simulink library "dspmathops"  (Simulink 8.0)
settings: Solver=ode45  SolverMode=SingleTasking  StartTime=0.0  StopTime=10.0  RelTol=1e-3
values from neighbouring files (symbols this model uses):
  D = D + B    [rebuffer_delay.m]
undefined symbols (not defined in the file or in its folder): dBval, Floor, fuzz_val, jsin, magnitude
libraries: dspsigattribs x2
settings Model: RequirementInfo=9  Creator=don  LastModifiedBy=lij  CovMetricSettings=d  ExtModeAutoUpdateStatusClock=off

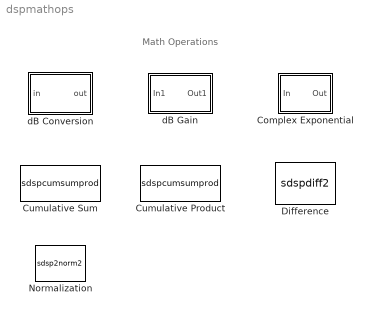
== system dspmathops ==
  note: Math Operations
  Complex Exponential : Subsystem
      mask Type: Complex Exponential
      mask Description:
      | Compute the complex exponential function of real inputs via
      | Euler's formula, y = cos(x)+jsin(x).
      mask Help: eval('blocksethelp');
      mask Display: text(0.2, 0.55,'exp(jx)');
  Cumulative Product : S-Function  DialogController=dspDDGCreate  DialogControllerArgs=DataTag1  FunctionName=sdspcumsumprod  Parameters=dim,InputProcessing,reset,fcn,outputMin,outputMax,dtInfo.interProdMode,dtInfo.interProdWordLength,dtInfo.interProdFracLength,dtInfo.prodOutputMode,dtInfo.prodOutputWordLength,dtInfo.prodOutputFracLength,dtInfo.accumMode,dtInfo.accumWordLength,dtInfo.accumFracLength,dtInfo.outputMode,dtInfo.outputWordLength,dtInfo.outputFracLength,dtInfo.roundingMode,dtInfo.overflowMode  EnableBusSupport=off  mask(Cumulative Product){dim=Channels (running product), InputProcessing=Columns as channels (frame based), reset_popup=None, interProdMode=Same as input, interProdWordLength=16, interProdFracLength=15, interProdDataTypeStr=Inherit: Same as input, interProdLastDataTypeStr=Inherit: Same as input, prodOutputMode=Same as input, prodOutputWordLength=32, prodOutputFracLength=30, prodOutputDataTypeStr=Inherit: Same as input, prodOutputLastDataTypeStr=Inherit: Same as input, accumMode=Same as input, accumWordLength=32, accumFracLength=30, accumDataTypeStr=Inherit: Same as input, accumLastDataTypeStr=Inherit: Same as input, outputMode=Same as input, outputWordLength=16, outputFracLength=15, outputDataTypeStr=Inherit: Same as input, outputLastDataTypeStr=Inherit: Same as input, outputMin=[], outputMax=[], roundingMode=Floor, overflowMode=off, LockScale=off}
      mask prompts: dim "Multiply input along:"; InputProcessing "Input processing:"; reset_popup "Reset port:"; interProdMode "inter prod mode"; interProdWordLength "inter prod wl"; interProdFracLength "inter prod fl"; interProdDataTypeStr "Intermediate product data type string:"; interProdLastDataTypeStr "Last intermediate product data type string:"; prodOutputMode "prod output mode"; prodOutputWordLength "prod output wl"; prodOutputFracLength "prod output fl"; prodOutputDataTypeStr "ProdOutput data type string:"; prodOutputLastDataTypeStr "Last prodOutput data type string:"; accumMode "accum mode"; accumWordLength "accum wl"; accumFracLength "accum fl"; accumDataTypeStr "Accum data type string:"; accumLastDataTypeStr "Last accum data type string:"; outputMode "output mode"; outputWordLength "output wl"; outputFracLength "output fl"; outputDataTypeStr "Output data type string:"; outputLastDataTypeStr "Last output data type string:"; outputMin "Output minimum:"; outputMax "Output maximum:"; roundingMode "rm"; overflowMode "om"; LockScale "Lock scaling"
      mask help: Cumulative product of input matrix or input vector elements along the specified dimension: rows, columns, or channels.
      mask init:
      | blkh   = gcbh;
      | reset  = reset_popup-1;
      | fcn    = 1;
      | dspSetFrameUpgradeParameter(blkh, 'InputProcessing', 'Inherited (this choice will be removed - see release notes)');
      | dtRows = dspblkGetCumProdDTRowInfo();
      | dtInfo = dspGetUDTFixptDataTypeInfo(blkh, dtRows, true);
      mask Help: eval('blocksethelp');
      mask StyleString: popup(Columns|Rows|Channels (running product)),popup(Columns as channels (frame based)|Elements as channels (sample based)|Inherited (this choice will be removed - see release notes)),popup(None|Rising edge|Falling edge|Either edge|Non-zero sample),popup(Same as input|Binary point scaling|Slope and bias scaling),edit,edit,unidt({a=7|||}{i=Inherit: Same as input}{s=UDTBinaryPointMode}{g=UDTInheritSign}),edit,popup(Same as input|Binary point scaling|Slope and bias scaling),edit,edit,unidt({a=12|||}{i=Inherit: Same as input}{s=UDTBinaryPointMode}{g=UDTInheritSign}),edit,popup(Same as product output|Same as input|Binary point scaling|Slope and bias scaling),edit,edit,unidt({a=17|||}{i=Inherit: Same as input|Inherit: Same as product output}{s=UDTBinaryPointMode}{g=UDTInheritSign}),edit,popup(Same as product output|Same as input|Binary point scaling|Slope and bias scaling),edit,edit,unidt({a=22|24|25|}{i=Inherit: Same as input|Inherit: Same as product output}{s=UDTBinaryPointMode}{g=UDTInheritSign}),edit,min,max,popup(Ceiling|Convergent|Floor|Nearest|Round|Simplest|Zero),checkbox,checkbox
      mask Display:
      | s = dspblkcumsumprod();
      | disp([s.str '\nProduct'])
      | port_label('input',s.i1,s.i1s);
      | port_label('input',s.i2,s.i2s);
  Cumulative Sum : S-Function  DialogController=dspDDGCreate  DialogControllerArgs=DataTag3  FunctionName=sdspcumsumprod  Parameters=dim,InputProcessing,reset,fcn,outputMin,outputMax,-1,0,0,-1,0,0,dtInfo.accumMode,dtInfo.accumWordLength,dtInfo.accumFracLength,dtInfo.outputMode,dtInfo.outputWordLength,dtInfo.outputFracLength,dtInfo.roundingMode,dtInfo.overflowMode  EnableBusSupport=off  mask(Cumulative Sum){dim=Channels (running sum), InputProcessing=Columns as channels (frame based), reset_popup=None, accumMode=Same as input, accumWordLength=32, accumFracLength=30, accumDataTypeStr=Inherit: Same as input, accumLastDataTypeStr=Inherit: Same as input, outputMode=Same as accumulator, outputWordLength=16, outputFracLength=15, outputDataTypeStr=Inherit: Same as accumulator, outputLastDataTypeStr=Inherit: Same as accumulator, outputMin=[], outputMax=[], roundingMode=Floor, overflowMode=off, LockScale=off}
      mask prompts: dim "Sum input along:"; InputProcessing "Input processing:"; reset_popup "Reset port:"; accumMode "accMode"; accumWordLength "accWL"; accumFracLength "accFL"; accumDataTypeStr "Accum data type string:"; accumLastDataTypeStr "Last accum data type string:"; outputWordLength "outputWL"; outputFracLength "outputFL"; outputDataTypeStr "Output data type string:"; outputLastDataTypeStr "Last output data type string:"; outputMin "Output minimum:"; outputMax "Output maximum:"; roundingMode "rm"; overflowMode "om"; LockScale "Lock scaling"
      mask help: Cumulative sum of input matrix or input vector elements along the specified dimension: rows, columns, or channels.
      mask init:
      | blkh   = gcbh;
      | reset  = reset_popup-1;
      | fcn    = 0;
      | dspSetFrameUpgradeParameter(blkh, 'InputProcessing', 'Inherited (this choice will be removed - see release notes)');
      | dtRows = dspblkGetCumSumDTRowInfo();
      | dtInfo = dspGetUDTFixptDataTypeInfo(blkh, dtRows, true);
      mask Help: eval('blocksethelp');
      mask StyleString: popup(Columns|Rows|Channels (running sum)),popup(Columns as channels (frame based)|Elements as channels (sample based)|Inherited (this choice will be removed - see release notes)),popup(None|Rising edge|Falling edge|Either edge|Non-zero sample),popup(Same as input|Binary point scaling|Slope and bias scaling),edit,edit,unidt({a=7|||}{i=Inherit: Same as input}{s=UDTBinaryPointMode}{g=UDTInheritSign}),edit,popup(Same as accumulator|Same as input|Binary point scaling|Slope and bias scaling),edit,edit,unidt({a=12|14|15|}{i=Inherit: Same as input|Inherit: Same as accumulator}{s=UDTBinaryPointMode}{g=UDTInheritSign}),edit,min,max,popup(Ceiling|Convergent|Floor|Nearest|Round|Simplest|Zero),checkbox,checkbox
      mask Display:
      | s = dspblkcumsumprod();
      | disp([s.str '\nSum'])
      | port_label('input',s.i1,s.i1s);
      | port_label('input',s.i2,s.i2s);
  Difference : S-Function  DialogController=dspDDGCreate  DialogControllerArgs=DataTag5  FunctionName=sdspdiff2  Parameters=Run,dim,Dimension,outputMin,outputMax,dtInfo.accumMode,dtInfo.accumWordLength,dtInfo.accumFracLength,dtInfo.outputMode,dtInfo.outputWordLength,dtInfo.outputFracLength,dtInfo.roundingMode,dtInfo.overflowMode  EnableBusSupport=off  mask(Difference){Run=No, dim=Columns, Dimension=1, additionalParams=off, allowOverrides=on, outputMode=Same as accumulator, outputWordLength=16, outputFracLength=15, outputDataTypeStr=Inherit: Same as accumulator, outputLastDataTypeStr=Inherit: Same as accumulator, outputMin=[], outputMax=[], accumMode=Inherit via internal rule, accumWordLength=32, accumFracLength=30, accumDataTypeStr=Inherit: Inherit via internal rule, accumLastDataTypeStr=Inherit: Inherit via internal rule, roundingMode=Floor, overflowMode=off, LockScale=off}
      mask prompts: Run "Running difference:"; dim "Difference along:"; additionalParams "------- Show additional parameters -------"; allowOverrides "Allow overrides from DSP Fixed-Point Attributes blocks"; outputMode "Fixed-point output attributes:"; outputWordLength "Output word length:"; outputFracLength "Output fraction length:"; outputDataTypeStr "Output data type string:"; outputLastDataTypeStr "Last output data type string:"; outputMin "Output minimum:"; outputMax "Output maximum:"; accumMode "Fixed-point accumulator attributes:"; accumWordLength "Accumulator word length:"; accumFracLength "Accumulator fraction length:"; accumDataTypeStr "Accum data type string:"; accumLastDataTypeStr "Last accum data type string:"; roundingMode "Round integer calculations toward:"; overflowMode "Saturate on integer overflow"; LockScale "Lock scaling"
      mask help: Difference between adjacent input elements. For oriented inputs, difference along the specified dimension.
      mask init:
      | blkh   = gcbh;
      | dspSetFrameUpgradeParameter(blkh, 'Run', 'Inherit from input (this choice will be removed - see release notes)');
      | dtRows = dspblkGetDiffDTRowInfo();
      | dtInfo = dspGetUDTFixptDataTypeInfo(blkh, dtRows, true);
      mask Help: eval('blocksethelp');
      mask StyleString: popup(No|Yes|Inherit from input (this choice will be removed - see release notes)),popup(Columns|Rows|Specified dimension),edit,checkbox,checkbox,popup(Same as accumulator|Same as input|Binary point scaling|Slope and bias scaling|User-defined),edit,edit,unidt({a=9|11|12|}{i=Inherit: Same as input|Inherit: Same as accumulator}{s=UDTBinaryPointMode}{g=UDTInheritSign}),edit,min,max,popup(Inherit via internal rule|Same as input|Binary point scaling|Slope and bias scaling|User-defined),edit,edit,unidt({a=16|||}{i=Inherit: Inherit via internal rule|Inherit: Same as input}{s=UDTBinaryPointMode}{g=UDTInheritSign}),edit,popup(Ceiling|Convergent|Floor|Nearest|Round|Simplest|Zero),checkbox,checkbox
      mask Display:
      | if strcmpi(get_param(gcbh, 'Run'), 'Yes')
      |     disp('Running\nDiff');
      | else
      |     disp('Diff');
      | end
  Normalization : S-Function  DialogController=dspDDGCreate  DialogControllerArgs=DataTag6  FunctionName=sdsp2norm2  Parameters=Bias,NormType,NormOver,ColComp,Dimension,outputMin,outputMax,dtInfo.prodOutputMode,dtInfo.prodOutputWordLength,dtInfo.prodOutputFracLength,dtInfo.accumMode,dtInfo.accumWordLength,dtInfo.accumFracLength,dtInfo.outputMode,dtInfo.outputWordLength,dtInfo.outputFracLength,dtInfo.roundingMode,dtInfo.overflowMode  EnableBusSupport=off  mask(Normalization){NormType=Squared 2-norm, Bias=1e-10, NormOver=Each column, ColComp=on, Dimension=1, additionalParams=off, allowOverrides=on, outputMode=Same as product output, outputWordLength=32, outputFracLength=32, outputDataTypeStr=Inherit: Same as product output, outputLastDataTypeStr=Inherit: Same as product output, outputMin=[], outputMax=[], accumMode=Same as product output, accumWordLength=32, accumFracLength=30, accumDataTypeStr=Inherit: Same as product output, accumLastDataTypeStr=Inherit: Same as product output, prodOutputMode=Same as input, prodOutputWordLength=32, prodOutputFracLength=32, prodOutputDataTypeStr=Inherit: Same as input, prodOutputLastDataTypeStr=Inherit: Same as input, roundingMode=Floor, overflowMode=off, LockScale=off}
      mask prompts: NormType "Norm:"; Bias "Normalization bias:"; NormOver "Normalize over:"; ColComp "Treat sample-based row input as a column"; additionalParams "--------------- Show additional parameters ---------------"; allowOverrides "Allow overrides from DSP Attributes blocks"; outputMode "Fixed-point output attributes:"; outputWordLength "Output word length:"; outputFracLength "Output fraction length:"; outputDataTypeStr "Output data type string:"; outputLastDataTypeStr "Last output data type string:"; outputMin "Output minimum:"; outputMax "Output maximum:"; accumMode "Fixed-point accumulator attributes"; accumWordLength "Accumulator word length:"; accumFracLength "Accumulator fraction length:"; accumDataTypeStr "Accum data type string:"; accumLastDataTypeStr "Last accum data type string:"; prodOutputMode "Fixed-point product output attributes:"; prodOutputWordLength "Product output word length:"; prodOutputFracLength "Product output fraction length:"; prodOutputDataTypeStr "ProdOutput data type string:"; prodOutputLastDataTypeStr "Last prodOutput data type string:"; roundingMode "Round integer calculations toward:"; overflowMode "Saturate on integer overflow"; LockScale "Lock scaling"
      mask help: Normalize the input over the specified dimension by the vector 2-norm, sqrt(u'u)+b, or by the squared 2-norm, u'u+b, where b is a bias used to protect against divide-by-zero. Normalization is performed over rows, columns, or the dimension of the input signal specified in the 'Dimension' parameter.
      mask init:
      | blkh   = gcbh;
      | dtRows = dspblkGetTwoNormDTRowInfo();
      | dtInfo = dspGetUDTFixptDataTypeInfo(blkh, dtRows, true);
      mask Help: eval('blocksethelp');
      mask StyleString: popup(2-norm|Squared 2-norm),edit,popup(Each column|Each row|Specified dimension),checkbox,edit,checkbox,checkbox,popup(Same as accumulator|Same as product output|Same as input|Binary point scaling|Slope and bias scaling),edit,edit,unidt({a=11|13|14|}{i=Inherit: Same as input|Inherit: Same as product output|Inherit: Same as accumulator}{s=UDTBinaryPointMode}{g=UDTInheritSign}),edit,min,max,popup(Same as product output|Same as input|Binary point scaling|Slope and bias scaling),edit,edit,unidt({a=18|||}{i=Inherit: Same as input|Inherit: Same as product output}{s=UDTBinaryPointMode}{g=UDTInheritSign}),edit,popup(Same as input|Binary point scaling|Slope and bias scaling),edit,edit,unidt({a=23|||}{i=Inherit: Same as input}{s=UDTBinaryPointMode}{g=UDTInheritSign}),edit,popup(Ceiling|Convergent|Floor|Nearest|Round|Simplest|Zero),checkbox,checkbox
      mask Display:
      | x = [0 NaN 100 NaN 20 80 NaN 30 30 NaN 36 36 NaN 58 58 NaN 64 64];
      | y = [0 NaN 100 NaN 60 60 NaN 9 43 NaN 9 43 NaN 9 43 NaN 9 43];
      | if NormType==1, sqr_txt = ' '; else sqr_txt = '2'; end
      | plot(x,y)
      | text(44,80,'u'); text(44,25,'u'); text(72,39,sqr_txt)
  dB Conversion : Subsystem  mask(dB Conversion){dBtype=dB, intype=Amplitude, R=1, fuzz=off}
      mask prompts: dBtype "Convert to:"; intype "Input signal:"; R "Load resistance (ohms):"; fuzz "Add eps to input to protect against  "log(0) = -inf""
      mask help: Convert input of watts or volts to decibels. Voltage inputs are first converted to power relative to the specified load resistance, where P = (V^2)/R. When converting to dB, the reference power is 1 W. When converting to dBm, the reference power is 1 mW.
      mask init:
      | [str fuzz_val dBval] = dspblkdb2('init');
      | dspblkdb2('checkparam');
      | dspblkdb2('update');
      mask Help: eval('blocksethelp');
      mask StyleString: popup(dB|dBm),popup(Power|Amplitude),edit,checkbox
      mask CallbackString: dspblkdb2|dspblkdb2||
      mask Display: disp(str)
  dB Gain : Subsystem  mask(dB Gain){dB=-40, intype=Amplitude}
      mask prompts: dB "Gain, dB:"; intype "Input signal:"
      mask help: Apply a gain specified in dB.
      mask init:
      | if isempty(dB)
      |   dB = 0; g = 0;
      |   s  = ['dB Gain'];
      | else
      |   g=10.^(dB/(10*intype));
      |   if (isscalar(dB))
      |     s = sprintf('%g dB\n(%g)',dB,g);
      |   else
      |     s = ['dB Gain'];
      |   end
      | end
      mask Help: eval('blocksethelp');
      mask StyleString: edit,popup(Power|Amplitude)
      mask Display: fprintf(s)

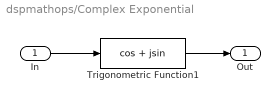
== system dspmathops/Complex Exponential ==
  In : Inport
  Trigonometric Function1 : Trigonometry  Operator=cos + jsin
  Out : Outport
  wires:
  Trigonometric Function1/1 -> Out/1
  In/1 -> Trigonometric Function1/1

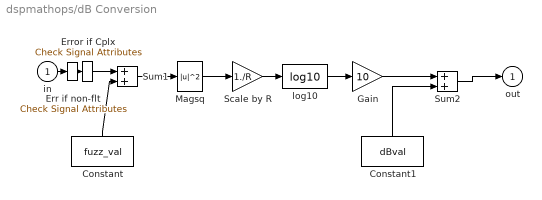
== system dspmathops/dB Conversion ==
  in : Inport
  Constant : Constant  Value=fuzz_val  OutDataTypeStr=Inherit: Inherit via back propagation
  Constant1 : Constant  Value=dBval  OutDataTypeStr=Inherit: Inherit via back propagation
  Err if non-flt : dspsigattribs/Check Signal Attributes  SystemSampleTime=-1  SigAttribCheckMethod=Does not match attributes exactly  Complexity=Ignore  Frame=Ignore  DimsCheckMethod=Ignore  Dimensions=1-D  DatatypeCheckMethod=Is...  DatatypeGeneral=Floating-point  DtypeFloatSpecific=Any floating-point  DtypeFixedSpecific=Any fixed-point  DtypeIntSpecific=Any integer  SampleMode=Ignore
  Error if Cplx : dspsigattribs/Check Signal Attributes  SystemSampleTime=-1  SigAttribCheckMethod=Matches attributes exactly  Complexity=Complex  Frame=Ignore  DimsCheckMethod=Ignore  Dimensions=1-D  DatatypeCheckMethod=Ignore  DatatypeGeneral=Boolean  DtypeFloatSpecific=Any floating-point  DtypeFixedSpecific=Any fixed-point  DtypeIntSpecific=Any integer  SampleMode=Ignore
  Gain : Gain  Gain=10  SaturateOnIntegerOverflow=on  OutDataTypeStr=Inherit: Same as input  ParamDataTypeStr=Inherit: Same as input
  Magsq : Math  Operator=magnitude^2  SaturateOnIntegerOverflow=on
  Scale by R : Gain  Gain=1./R  SaturateOnIntegerOverflow=on  OutDataTypeStr=Inherit: Same as input  ParamDataTypeStr=Inherit: Same as input
  Sum1 : Sum  SaturateOnIntegerOverflow=on  InputSameDT=on  OutDataTypeStr=Inherit: Same as first input
  Sum2 : Sum  SaturateOnIntegerOverflow=on  InputSameDT=on  OutDataTypeStr=Inherit: Same as first input
  log10 : Math  Operator=log10  SaturateOnIntegerOverflow=on
  out : Outport  InitialOutput=0
  wires:
  Constant1/1 -> Sum2/2
  Sum2/1 -> out/1
  Gain/1 -> Sum2/1
  Constant/1 -> Sum1/2
  Sum1/1 -> Magsq/1
  Error if Cplx/1 -> Sum1/1
  in/1 -> Err if non-flt/1
  Err if non-flt/1 -> Error if Cplx/1
  Scale by R/1 -> log10/1
  Magsq/1 -> Scale by R/1
  log10/1 -> Gain/1

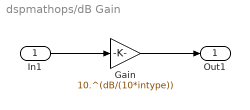
== system dspmathops/dB Gain ==
  In1 : Inport
  Gain : Gain  Gain=10.^(dB/(10*intype))
  Out1 : Outport
  wires:
  In1/1 -> Gain/1
  Gain/1 -> Out1/1
